simulink model "modeloIntegrador2015"  (R2015b)
settings: Solver=ode45  StartTime=0.0  StopTime=10  MaxStep=1e-3  RelTol=1e-3
undefined symbols (not defined in the file or in its folder): Kenc, Km, Ktac, taum
settings Model: Creator=03135  LastModifiedBy=LucasSerrano
settings DataIOCC: SaveFormat=Array  SignalLoggingSaveFormat=ModelDataLogs
settings OptimizationCC: ExpressionDepthLimit=2147483647
settings DebuggingCC: UnderspecifiedInitializationDetection=Classic  MergeDetectMultiDrivingBlocksExec=none  SolverPrmCheckMsg=warning  FcnCallInpInsideContextMsg=UseLocalSettings  AllowSymbolicDim=on  StateNameClashWarn=warning
settings HardwareCC: ProdBitPerPointer=32  ProdLargestAtomicFloat=None  ProdIntDivRoundTo=Undefined  ProdEndianess=Unspecified  ProdWordSize=32  ProdHWDeviceType=32-bit Generic
settings GRTTargetCC: GeneratePreprocessorConditionals=Disable all  CombineOutputUpdateFcns=off  GRTInterface=on
settings ConfigComp: CovModelRefEnable=Off

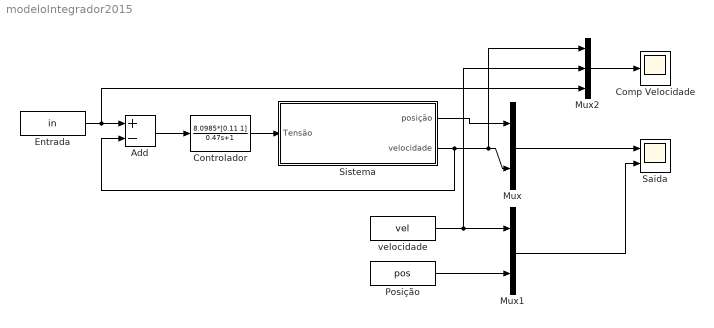
== system modeloIntegrador2015 ==
  Add : Sum  Inputs=+-
  Comp Velocidade : Scope
  Controlador : TransferFcn  Numerator=8.0985*[0.11 1]  Denominator=[0.47 1]
  Entrada : FromWorkspace  VariableName=in  SampleTime=0
  Mux : Mux  Inputs=2
  Mux1 : Mux  Inputs=2
  Mux2 : Mux  Inputs=3
  Posição : FromWorkspace  VariableName=pos  SampleTime=0
  Saida : Scope  NumInputPorts=2
  Sistema : Subsystem
  velocidade : FromWorkspace  VariableName=vel  SampleTime=0
  wires:
  Mux/1 -> Saida/1
  Sistema/1(posição) -> Mux/1
  Sistema/2(velocidade) -> Add/2, Mux2/1, Mux/2
  Mux1/1 -> Saida/2
  velocidade/1 -> Mux2/2, Mux1/1
  Posição/1 -> Mux1/2
  Mux2/1 -> Comp Velocidade/1
  Entrada/1 -> Mux2/3, Add/1
  Add/1 -> Controlador/1
  Controlador/1 -> Sistema/1(Tensão)

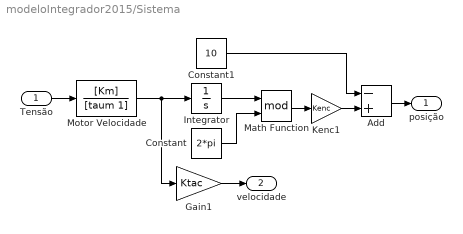
== system modeloIntegrador2015/Sistema ==
  Tensão : Inport
  Add : Sum  Inputs=-+
  Constant : Constant  Value=2*pi
  Constant1 : Constant  Value=10
  Gain1 : Gain  Gain=Ktac
  Integrator : Integrator
  Kenc1 : Gain  Gain=Kenc
  Math Function : Math  Operator=mod  SaturateOnIntegerOverflow=on
  Motor Velocidade : TransferFcn  Numerator=[Km]  Denominator=[taum 1]
  posição : Outport
  velocidade : Outport  Port=2
  wires:
  Motor Velocidade/1 -> Integrator/1, Gain1/1
  Tensão/1 -> Motor Velocidade/1
  Gain1/1 -> velocidade/1
  Math Function/1 -> Kenc1/1
  Integrator/1 -> Math Function/1
  Constant/1 -> Math Function/2
  Add/1 -> posição/1
  Kenc1/1 -> Add/2
  Constant1/1 -> Add/1
